simulink model "Wind_turbin."  (R2022b)
settings: Solver=ode45  StartTime=0.0  StopTime=Tsim  FixedStep=5e-5  RelTol=1e-6  EnableMultiTasking=on
values from neighbouring files (symbols this model uses):
  c1 = 0.44    [wind_code.m]
  c2 = 125    [wind_code.m]
  c3 = 0    [wind_code.m]
  c4 = 0    [wind_code.m]
  c5 = 0    [wind_code.m]
  c6 = 6.94    [wind_code.m]
  c7 = 16.5    [wind_code.m]
  c8 = 0    [wind_code.m]
  c9 = -0.002    [wind_code.m]
  N = 80    [wind_code.m]
  p = 2    [wind_code.m]
undefined symbols (not defined in the file or in its folder): A, Cdc, f_n1, fluxm, Jtot, Kcp, ki_dc, ki_m, ki_P_n1, ki_pll_n1, ki_s_n1, kp_dc, kp_md, kp_mq, kp_P_n1, kp_pll_n1, kp_s_n1, Lc_n1, Ld, Lg_n1, Lq, magnitud_delay, pitch, Q_set, Rc_n1, Rg_n1, rho, Rs, Rt, t_step_Q, Vdcref_n1, Vpeak_n1, w_n1
libraries: spsControlledVoltageSourceLib x9, slpidlib x8, spsSeriesRLCBranchLib x7, spsCurrentMeasurementLib x3, spsGroundLib x2, spsThreePhaseVIMeasurementLib x2, spsControlledCurrentSourceLib x2, spsPower3phInstantaneousLib x2, spsPermanentMagnetSynchronousMachineLib x1, spsVoltageMeasurementLib x1, sps_lib x1
(part 1 of 2)
settings Model: ExtModeTrigDuration=100  Creator=Enric  LastModifiedBy=Admin
settings SolverCC: SolverJacobianMethodControl=FullPerturbation  AlgebraicLoopSolver=TrustRegion
settings DataIOCC: LimitDataPoints=on  SaveOutput=off  ReturnWorkspaceOutputs=off  StateSaveName=tmp_raccel_xout  SignalLoggingName=tmp_raccel_logsout
settings OptimizationCC: ReuseModelBlockBuffer=on  EfficientMapNaN2IntZero=off  LifeSpan=inf
settings DebuggingCC: UnconnectedInputMsg=warning  UnconnectedOutputMsg=warning  UnconnectedLineMsg=warning  AllowSymbolicDim=off  SFUnexpectedBacktrackingDiag=warning  SFNoUnconditionalDefaultTransitionDiag=warning  SFExecutionAtInitializationDiag=none  ArithmeticOperatorsInVariantConditions=warning
settings HardwareCC: TargetBitPerPointer=64  TargetBitPerSizeT=64  TargetBitPerPtrDiffT=64  TargetLongLongMode=on  TargetIntDivRoundTo=Zero  TargetEndianess=LittleEndian  TargetWordSize=64  TargetHWDeviceType=MATLAB Host  ProdEqTarget=off
settings ModelReferenceCC: EnableRefExpFcnMdlSchedulingChecks=on  PropagateSignalLabelsOutOfModel=off
settings SFSimCC: SimUseLocalCustomCode=off  CustomCodeUndefinedFunction=UseInterfaceOnly
settings RTWCC: SystemTargetFile=raccel.tlc  TemplateMakefile=raccel_default_tmf  RTWVerbose=off  RTWUseLocalCustomCode=off  RTWUseSimCustomCode=on  DLArmComputeVersion=19.05
settings CodeAppCC: GenerateComments=off  MaxIdLength=128  MangleLength=10  SimulinkBlockComments=off
settings RaccelTargetCC: OptimizeReductions=off  ENABLE_SLEXEC_SSBRIDGE=0  RTWCAPISignals=off  RTWCAPIParams=on  RTWCAPIRootIO=off
settings ConfigComp: CovMetricSettings=dw  CovSaveCumulativeToWorkspaceVar=on  CovSaveSingleToWorkspaceVar=on  CovExternalEMLEnable=off
settings SimscapeCC: SimscapeNormalizeSystem=off

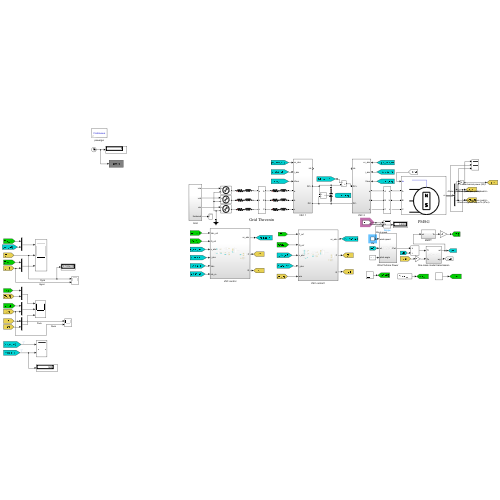
[thumbnail: Simulink's stored preview of the top-level diagram]
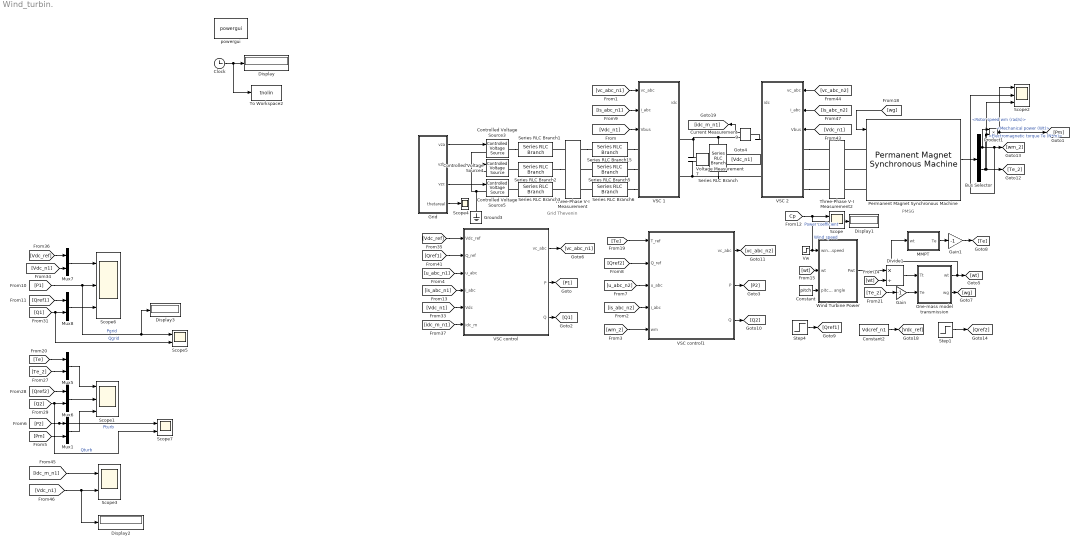
== system Wind_turbin. ==
  note: Grid Thevenin
  note: PMSG
  Bus Selector : BusSelector  OutputSignals=Rotor speed wm (rad/s),Electromagnetic torque Te (N*m)
  Clock : Clock
  Constant : Constant  Value=pitch
  Constant2 : Constant  Value=Vdcref_n1
  Controlled Voltage Source3 : spsControlledVoltageSourceLib/Controlled Voltage Source  Initialize=off  Source_Type=AC  Amplitude=0  Phase=0  Frequency=0  Measurements=None
  Controlled Voltage Source4 : spsControlledVoltageSourceLib/Controlled Voltage Source  Initialize=off  Source_Type=AC  Amplitude=0  Phase=0  Frequency=0  Measurements=None
  Controlled Voltage Source5 : spsControlledVoltageSourceLib/Controlled Voltage Source  Initialize=off  Source_Type=AC  Amplitude=0  Phase=0  Frequency=0  Measurements=None
  Current Measurement9 : spsCurrentMeasurementLib/Current Measurement  PhasorSimulation=off  OutputType=Complex  PSBequivalent=0
  Display{,1..3} (4 alike) : Display
  Divide1 : Product  Inputs=*/
  Gain : Gain  Gain=-1
  Gain1 : Gain  Gain=-1
  Grid : Subsystem
  Ground3 : spsGroundLib/Ground  LConnTagsString=a
  MMPT : Subsystem
  Mux{1,5..8} (5 alike) : Mux  Inputs=2
  One-mass model transmission : Subsystem
  Permanent Magnet Synchronous Machine : spsPermanentMagnetSynchronousMachineLib/Permanent Magnet Synchronous Machine  NbPhases=3  FluxDistribution=Sinusoidal  RotorType=Round  MechanicalLoad=Speed w  PresetModel=No  ShowDetailedParameters=on  MeasurementBus=off  Resistance=Rs  Inductance=8.5e-3  dqInductances=[Ld,Lq]  La=Lqd  MachineConstant=Flux linkage established by magnets (V.s)  Flux=fluxm  VoltageCst=906.8997  TorqueCst=7.5  Flat=120  Mechanical=[0.0027 0 1 0]  PolePairs=p  InitialConditions=[w_n1/p,0, 0,0]  InitialConditions5ph=[0 0 0 0 0 0]  RefAngle=90 degrees behind phase A axis (modified Park)  IterativeDiscreteModel=Trapezoidal non iterative  TsBlock=-1  TsPowergui=0
  Product1 : Product
  Scope{,3,5,7} (4 alike) : Scope  NumInputPorts=2
  Scope1 : Scope  NumInputPorts=3
  Scope2 : Scope  NumInputPorts=3
  Scope4 : Scope
  Scope6 : Scope  NumInputPorts=3
  Series RLC Branch : spsSeriesRLCBranchLib/Series RLC Branch  LConnTagsString=__new0  RConnTagsString=__new0  BranchType=C  Resistance=1  Inductance=1e-3  SetiL0=off  InitialCurrent=0  Capacitance=Cdc  Setx0=on  InitialVoltage=Vdcref_n1  Measurements=None
  Series RLC Branch1 : spsSeriesRLCBranchLib/Series RLC Branch  LConnTagsString=__new0  RConnTagsString=__new0  BranchType=RL  Resistance=Rg_n1  Inductance=Lg_n1  SetiL0=off  InitialCurrent=0  Capacitance=0  Setx0=off  InitialVoltage=0  Measurements=None
  Series RLC Branch15 : spsSeriesRLCBranchLib/Series RLC Branch  LConnTagsString=__new0  RConnTagsString=__new0  BranchType=RL  Resistance=Rc_n1  Inductance=Lc_n1  SetiL0=off  InitialCurrent=0  Capacitance=0  Setx0=off  InitialVoltage=0  Measurements=None
  Series RLC Branch2 : spsSeriesRLCBranchLib/Series RLC Branch  LConnTagsString=__new0  RConnTagsString=__new0  BranchType=RL  Resistance=Rg_n1  Inductance=Lg_n1  SetiL0=off  InitialCurrent=0  Capacitance=0  Setx0=off  InitialVoltage=0  Measurements=None
  Series RLC Branch3 : spsSeriesRLCBranchLib/Series RLC Branch  LConnTagsString=__new0  RConnTagsString=__new0  BranchType=RL  Resistance=Rg_n1  Inductance=Lg_n1  SetiL0=off  InitialCurrent=0  Capacitance=0  Setx0=off  InitialVoltage=0  Measurements=None
  Series RLC Branch5 : spsSeriesRLCBranchLib/Series RLC Branch  LConnTagsString=__new0  RConnTagsString=__new0  BranchType=RL  Resistance=Rc_n1  Inductance=Lc_n1  SetiL0=off  InitialCurrent=0  Capacitance=0  Setx0=off  InitialVoltage=0  Measurements=None
  Series RLC Branch6 : spsSeriesRLCBranchLib/Series RLC Branch  LConnTagsString=__new0  RConnTagsString=__new0  BranchType=RL  Resistance=Rc_n1  Inductance=Lc_n1  SetiL0=off  InitialCurrent=0  Capacitance=0  Setx0=off  InitialVoltage=0  Measurements=None
  Step1 : Step  Time=t_step_Q  After=0  SampleTime=0
  Step4 : Step  Time=t_step_Q  Before=Q_set  After=Q_set*1.2  SampleTime=0
  Three-Phase V-I Measurement : spsThreePhaseVIMeasurementLib/Three-Phase V-I Measurement  VoltageMeasurement=phase-to-ground  SetLabelV=on  LabelV=u_abc_n1  Vpu=off  VpuLL=off  CurrentMeasurement=yes  SetLabelI=on  LabelI=is_abc_n1  Ipu=off  Pbase=100e6  Vbase=500e3  OutputType=Complex  PhasorSimulation=off  PSBequivalent=0
  Three-Phase V-I Measurement2 : spsThreePhaseVIMeasurementLib/Three-Phase V-I Measurement  VoltageMeasurement=phase-to-ground  SetLabelV=on  LabelV=u_abc_n2  Vpu=off  VpuLL=off  CurrentMeasurement=yes  SetLabelI=on  LabelI=is_abc_n2  Ipu=off  Pbase=100e6  Vbase=500e3  OutputType=Complex  PhasorSimulation=off  PSBequivalent=0
  To Workspace2 : ToWorkspace  VariableName=tnolin  SampleTime=-1
  VSC 1 : Subsystem
  VSC 2 : Subsystem
  VSC control : Subsystem
  VSC control1 : Subsystem
  Voltage Measurement7 : spsVoltageMeasurementLib/Voltage Measurement  PhasorSimulation=off  OutputType=Complex  PSBequivalent=0
  Vw : Step  Time=0.5  Before=5  After=8  SampleTime=0
  Wind Turbine Power : Subsystem
  powergui : sps_lib/powergui  Priority=1  SimulationMode=Continuous  SampleTime=1e-5  frequency=60  Iterations=50  frequencyindice=0  Pbase=100e6  ErrMax=1e-4  UnitsV=kV  UnitsW=MW  buscounter=0  FunctionMessages=off  echomessages=off  EnableUseOfTLC=off  CurrentSourceSwitches=off  DisableSnubberDevices=off  DisableRonSwitches=off  DisableVfSwitches=off  DisplayEquations=off  AutomaticDiscreteSolvers=off  SolverType=Tustin  Interpol=off  ExternalGateDelay=off  methode=off  Ts=0  x0status=blocks  SPID=off  SwTol=0  HookPort=off  NonlinearTolerance=1e-4  nMaxIteration=100  ContinueOnMaxIteration=off  RestoreLinks=warning  ResistiveCurrentMeasurement=off  Frange=[0:2:500]  Ylog=off  Xlog=on  ShowGrid=off  save=off  variable=ZData  structure=Vk  ZoomFFT=off  StartTime=2.01  cycles=3  DisplayStyle=1  fundamental=50  FreqAxis=off  MaxFrequency=1000  frequencyindicesteady=1  RmsSteady=1  display=off
  wires:
  Clock/1 -> To Workspace2/1, Display/1
  [Vdc_n1] -> VSC 1/3(Vbus)
  [is_abc_n1] -> VSC 1/2(i_abc)
  [vc_abc_n1] -> VSC 1/1(vc_abc)
  Voltage Measurement7/1 -> [Vdc_n1]
  Grid/1(vza) -> Controlled Voltage Source3/1
  Grid/3(vzc) -> Controlled Voltage Source5/1
  Grid/4(thetareal) -> Scope4/1
  Grid/2(vzb) -> Controlled Voltage Source4/1
  Step4/1 -> [Qref1]
  Mux6/1 -> Scope1/2
  Mux5/1 -> Scope1/1
  [Qref2] -> Mux6/1
  [Te_2] -> Mux5/2
  [Q2] -> Scope7/2, Mux6/2  "Qturb"
  [Vdc_n1] -> Mux7/2
  [Vdc_ref] -> Mux7/1
  Mux7/1 -> Scope6/1
  [P1] -> Display3/1, Scope5/1, Scope6/2  "Pgrid"
  [Q1] -> Scope5/2, Mux8/2  "Qgrid"
  [Qref1] -> Mux8/1
  Mux8/1 -> Scope6/3
  Current Measurement9/1 -> [idc_m_n1]
  [idc_m_n1] -> Scope3/1
  [Vdc_n1] -> Display2/1, Scope3/2
  Constant2/1 -> [Vdc_ref]
  Permanent Magnet Synchronous Machine/1 -> Bus Selector/1
  Bus Selector/1 -> Scope2/2, [wm_2], Product1/1  "<Rotor speed wm (rad/s)>"
  Bus Selector/2 -> [Te_2], Scope2/3, Product1/2  "<Electromagnetic torque Te (N*m)>"
  [Vdc_n1] -> VSC 2/3(Vbus)
  [is_abc_n2] -> VSC 2/2(i_abc)
  [vc_abc_n2] -> VSC 2/1(vc_abc)
  [Vdc_ref] -> VSC control/1(Vdc_ref)
  [Qref1] -> VSC control/2(Q_ref)
  VSC control/1(vc_abc) -> [vc_abc_n1]
  [u_abc_n1] -> VSC control/3(u_abc)
  [is_abc_n1] -> VSC control/4(i_abc)
  [Vdc_n1] -> VSC control/5(Vdc)
  [idc_m_n1] -> VSC control/6(idc_m)
  VSC control/2(P) -> [P1]
  VSC control/3(Q) -> [Q1]
  [is_abc_n2] -> VSC control1/4(i_abc)
  [u_abc_n2] -> VSC control1/3(u_abc)
  [Qref2] -> VSC control1/2(Q_ref)
  VSC control1/3(Q) -> [Q2]
  VSC control1/1(vc_abc) -> [vc_abc_n2]
  VSC control1/2(P) -> [P2]
  [wm_2] -> VSC control1/5(wm)
  Product1/1 -> Scope2/1, [Pm]  "<Mechanical power (Wt)>"
  [Pm] -> Mux1/2
  Mux1/1 -> Scope1/3
  [P2] -> Scope7/1, Mux1/1  "Pturb"
  One-mass model transmission/2(wg) -> [wg]
  [wt] -> Wind Turbine Power/2(wt)
  Wind Turbine Power/1(Pwt) -> Divide1/1
  One-mass model transmission/1(wt) -> MMPT/1(wt), [wt]
  MMPT/1(Te) -> Gain1/1
  [wt] -> Divide1/2
  Constant/1 -> Wind Turbine Power/3(pitch angle)
  Divide1/1 -> One-mass model transmission/1(Tt)
  Gain/1 -> One-mass model transmission/2(Te)
  [Te_2] -> Gain/1
  [wg] -> Permanent Magnet Synchronous Machine/1
  Vw/1 -> Scope/2, Wind Turbine Power/1(wind speed)  "Wind speed"
  [Te] -> VSC control1/1(T_ref)
  Gain1/1 -> [Te]
  [Te] -> Mux5/1
  Step1/1 -> [Qref2]
  [Cp] -> Display1/1, Scope/1  "Power coefficient"
  connections:
  Series RLC Branch6/RConn1 -- VSC 1/LConn3
  Series RLC Branch15/RConn1 -- VSC 1/LConn1
  Series RLC Branch5/RConn1 -- VSC 1/LConn2
  Three-Phase V-I Measurement/LConn1 -- Series RLC Branch15/LConn1
  Series RLC Branch6/LConn1 -- Three-Phase V-I Measurement/LConn3
  Series RLC Branch5/LConn1 -- Three-Phase V-I Measurement/LConn2
  Controlled Voltage Source5/LConn1 -- Ground3/LConn1 -- Controlled Voltage Source3/LConn1 -- Controlled Voltage Source4/LConn1
  Controlled Voltage Source3/RConn1 -- Series RLC Branch1/LConn1
  Series RLC Branch2/LConn1 -- Controlled Voltage Source4/RConn1
  Series RLC Branch3/LConn1 -- Controlled Voltage Source5/RConn1
  Three-Phase V-I Measurement/RConn3 -- Series RLC Branch3/RConn1
  Voltage Measurement7/LConn1 -- Current Measurement9/RConn1 -- Series RLC Branch/LConn1 -- VSC 1/RConn1
  Voltage Measurement7/LConn2 -- VSC 2/RConn2 -- Series RLC Branch/RConn1 -- VSC 1/RConn2
  Series RLC Branch2/RConn1 -- Three-Phase V-I Measurement/RConn2
  Three-Phase V-I Measurement/RConn1 -- Series RLC Branch1/RConn1
  VSC 2/LConn1 -- Three-Phase V-I Measurement2/LConn1
  VSC 2/LConn2 -- Three-Phase V-I Measurement2/LConn2
  VSC 2/LConn3 -- Three-Phase V-I Measurement2/LConn3
  Permanent Magnet Synchronous Machine/LConn1 -- Three-Phase V-I Measurement2/RConn1
  Permanent Magnet Synchronous Machine/LConn2 -- Three-Phase V-I Measurement2/RConn2
  Permanent Magnet Synchronous Machine/LConn3 -- Three-Phase V-I Measurement2/RConn3
  VSC 2/RConn1 -- Current Measurement9/LConn1

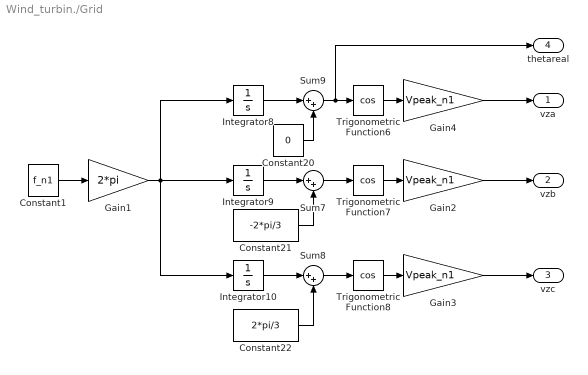
== system Wind_turbin./Grid ==
  Constant1 : Constant  Value=f_n1
  Constant20 : Constant  Value=0
  Constant21 : Constant  Value=-2*pi/3
  Constant22 : Constant  Value=2*pi/3
  Gain1 : Gain  Gain=2*pi
  Gain2 : Gain  Gain=Vpeak_n1
  Gain3 : Gain  Gain=Vpeak_n1
  Gain4 : Gain  Gain=Vpeak_n1
  Integrator10 : Integrator
  Integrator8 : Integrator
  Integrator9 : Integrator
  Sum7 : Sum  Inputs=|++
  Sum8 : Sum  Inputs=|++
  Sum9 : Sum  Inputs=|++
  Trigonometric Function6 : Trigonometry  Operator=cos
  Trigonometric Function7 : Trigonometry  Operator=cos
  Trigonometric Function8 : Trigonometry  Operator=cos
  vza : Outport
  vzb : Outport  Port=2
  vzc : Outport  Port=3
  thetareal : Outport  Port=4
  wires:
  Trigonometric Function7/1 -> Gain2/1
  Trigonometric Function8/1 -> Gain3/1
  Constant1/1 -> Gain1/1
  Sum9/1 -> thetareal/1, Trigonometric Function6/1
  Constant22/1 -> Sum8/2
  Integrator10/1 -> Sum8/1
  Constant21/1 -> Sum7/2
  Integrator8/1 -> Sum9/1
  Gain1/1 -> Integrator8/1, Integrator9/1, Integrator10/1
  Sum7/1 -> Trigonometric Function7/1
  Constant20/1 -> Sum9/2
  Trigonometric Function6/1 -> Gain4/1
  Integrator9/1 -> Sum7/1
  Sum8/1 -> Trigonometric Function8/1
  Gain4/1 -> vza/1
  Gain2/1 -> vzb/1
  Gain3/1 -> vzc/1

== system Wind_turbin./MMPT ==
  wt : Inport
  Gain6 : Gain  Gain=Kcp/N
  Product : Product
  Te : Outport
  wires:
  Product/1 -> Gain6/1
  wt/1 -> Product/1, Product/2
  Gain6/1 -> Te/1

== system Wind_turbin./One-mass model transmission ==
  Tt : Inport
  Te : Inport  Port=2
  Gain2 : Gain  Gain=N
  Gain3 : Gain  Gain=1/Jtot
  Gain4 : Gain  Gain=N
  Integrator : Integrator  InitialCondition=1
  Sum : Sum  Inputs=+-
  wt : Outport
  wg : Outport  Port=2
  wires:
  Gain4/1 -> wg/1
  Sum/1 -> Gain3/1
  Integrator/1 -> Gain4/1, wt/1
  Tt/1 -> Sum/1
  Gain3/1 -> Integrator/1
  Gain2/1 -> Sum/2
  Te/1 -> Gain2/1

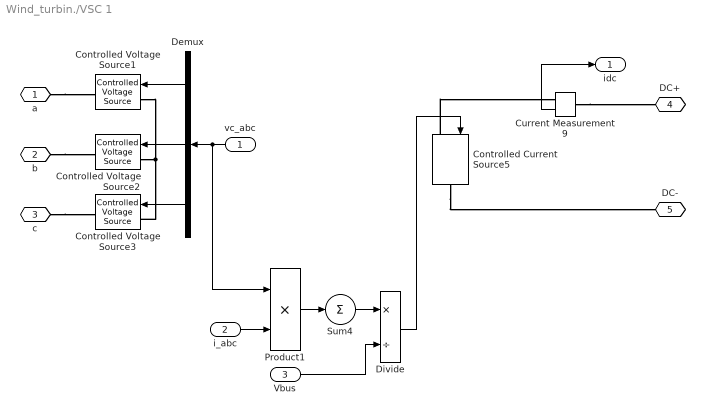
== system Wind_turbin./VSC 1 ==
  vc_abc : Inport
  i_abc : Inport  Port=2
  Vbus : Inport  Port=3
  Controlled Current Source5 : spsControlledCurrentSourceLib/Controlled Current Source  Initialize=on  Source_Type=DC  Amplitude=0  Phase=0  Frequency=0  Measurements=None
  Controlled Voltage Source1 : spsControlledVoltageSourceLib/Controlled Voltage Source  Initialize=off  Source_Type=AC  Amplitude=0  Phase=0  Frequency=0  Measurements=None
  Controlled Voltage Source2 : spsControlledVoltageSourceLib/Controlled Voltage Source  Initialize=off  Source_Type=AC  Amplitude=0  Phase=0  Frequency=0  Measurements=None
  Controlled Voltage Source3 : spsControlledVoltageSourceLib/Controlled Voltage Source  Initialize=off  Source_Type=AC  Amplitude=0  Phase=0  Frequency=0  Measurements=None
  Current Measurement9 : spsCurrentMeasurementLib/Current Measurement  PhasorSimulation=off  OutputType=Complex  PSBequivalent=0
  Demux : Demux  Outputs=3
  Divide : Product  Inputs=*/
  Product1 : Product  InputSameDT=on  SaturateOnIntegerOverflow=on  OutDataTypeStr=Inherit: Same as first input
  Sum4 : Sum  Inputs=1  InputSameDT=on  SaturateOnIntegerOverflow=on  OutDataTypeStr=Inherit: Same as first input
  a : PMIOPort  Side=Left
  b : PMIOPort  Port=2  Side=Left
  c : PMIOPort  Port=3  Side=Left
  DC+ : PMIOPort  Port=4  Side=Right
  DC- : PMIOPort  Port=5  Side=Right
  idc : Outport
  wires:
  Current Measurement9/1 -> idc/1
  Product1/1 -> Sum4/1
  Sum4/1 -> Divide/1
  Divide/1 -> Controlled Current Source5/1
  i_abc/1 -> Product1/2
  Demux/2 -> Controlled Voltage Source2/1
  Demux/1 -> Controlled Voltage Source1/1
  Demux/3 -> Controlled Voltage Source3/1
  vc_abc/1 -> Product1/1, Demux/1
  Vbus/1 -> Divide/2
  connections:
  Controlled Current Source5/RConn1 -- DC-/RConn1
  Controlled Current Source5/LConn1 -- Current Measurement9/RConn1
  Current Measurement9/LConn1 -- DC+/RConn1
  Controlled Voltage Source1/LConn1 -- Controlled Voltage Source2/LConn1 -- Controlled Voltage Source3/LConn1
  a/RConn1 -- Controlled Voltage Source1/RConn1
  b/RConn1 -- Controlled Voltage Source2/RConn1
  c/RConn1 -- Controlled Voltage Source3/RConn1

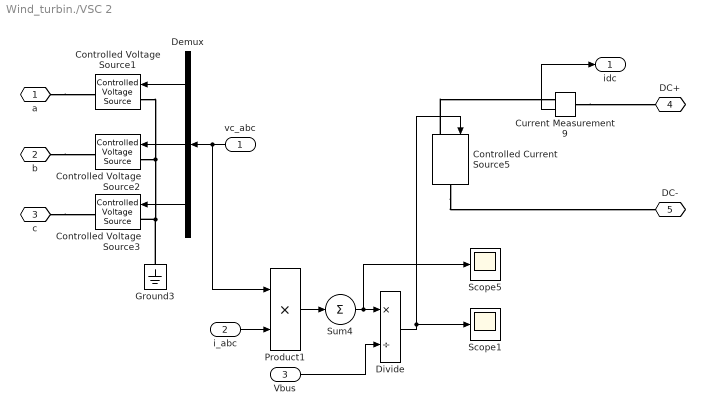
== system Wind_turbin./VSC 2 ==
  vc_abc : Inport
  i_abc : Inport  Port=2
  Vbus : Inport  Port=3
  Controlled Current Source5 : spsControlledCurrentSourceLib/Controlled Current Source  Initialize=on  Source_Type=DC  Amplitude=0  Phase=0  Frequency=0  Measurements=None
  Controlled Voltage Source1 : spsControlledVoltageSourceLib/Controlled Voltage Source  Initialize=off  Source_Type=AC  Amplitude=0  Phase=0  Frequency=0  Measurements=None
  Controlled Voltage Source2 : spsControlledVoltageSourceLib/Controlled Voltage Source  Initialize=off  Source_Type=AC  Amplitude=0  Phase=0  Frequency=0  Measurements=None
  Controlled Voltage Source3 : spsControlledVoltageSourceLib/Controlled Voltage Source  Initialize=off  Source_Type=AC  Amplitude=0  Phase=0  Frequency=0  Measurements=None
  Current Measurement9 : spsCurrentMeasurementLib/Current Measurement  PhasorSimulation=off  OutputType=Complex  PSBequivalent=0
  Demux : Demux  Outputs=3
  Divide : Product  Inputs=*/
  Ground3 : spsGroundLib/Ground  LConnTagsString=a
  Product1 : Product  InputSameDT=on  SaturateOnIntegerOverflow=on  OutDataTypeStr=Inherit: Same as first input
  Scope1 : Scope
  Scope5 : Scope
  Sum4 : Sum  Inputs=1  InputSameDT=on  SaturateOnIntegerOverflow=on  OutDataTypeStr=Inherit: Same as first input
  a : PMIOPort  Side=Left
  b : PMIOPort  Port=2  Side=Left
  c : PMIOPort  Port=3  Side=Left
  DC+ : PMIOPort  Port=4  Side=Right
  DC- : PMIOPort  Port=5  Side=Right
  idc : Outport
  wires:
  Current Measurement9/1 -> idc/1
  Product1/1 -> Sum4/1
  Sum4/1 -> Scope5/1, Divide/1
  Divide/1 -> Scope1/1, Controlled Current Source5/1
  i_abc/1 -> Product1/2
  Demux/2 -> Controlled Voltage Source2/1
  Demux/1 -> Controlled Voltage Source1/1
  Demux/3 -> Controlled Voltage Source3/1
  vc_abc/1 -> Product1/1, Demux/1
  Vbus/1 -> Divide/2
  connections:
  Controlled Current Source5/RConn1 -- DC-/RConn1
  Controlled Current Source5/LConn1 -- Current Measurement9/RConn1
  Current Measurement9/LConn1 -- DC+/RConn1
  Controlled Voltage Source1/LConn1 -- Controlled Voltage Source2/LConn1 -- Ground3/LConn1 -- Controlled Voltage Source3/LConn1
  a/RConn1 -- Controlled Voltage Source1/RConn1
  b/RConn1 -- Controlled Voltage Source2/RConn1
  c/RConn1 -- Controlled Voltage Source3/RConn1

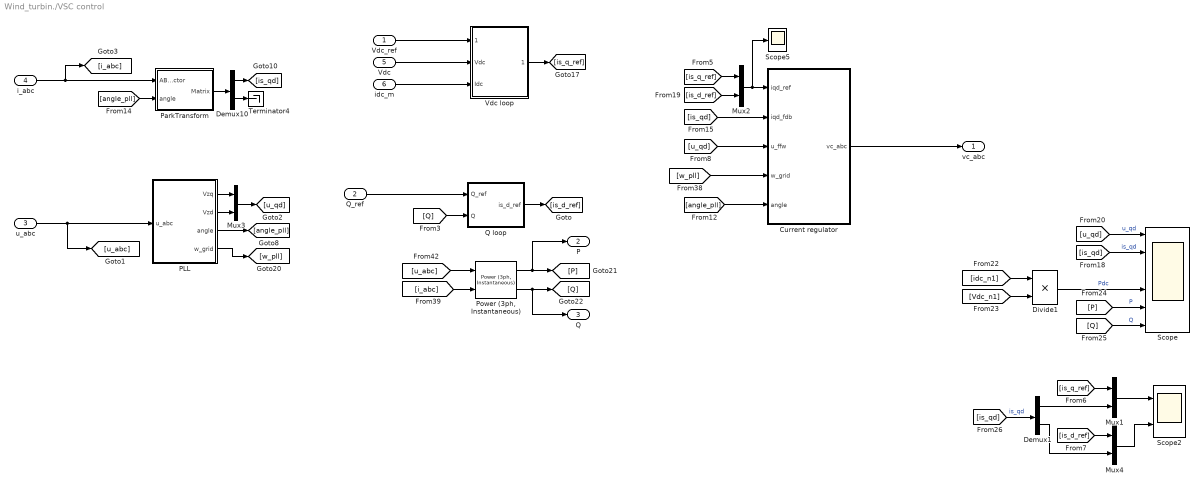
== system Wind_turbin./VSC control ==
  Vdc_ref : Inport
  Q_ref : Inport  Port=2
  u_abc : Inport  Port=3
  i_abc : Inport  Port=4
  Vdc : Inport  Port=5
  idc_m : Inport  Port=6
  Current regulator : Subsystem
  Demux1 : Demux  Outputs=2
  Demux10 : Demux  Outputs=2
  Divide1 : Product  Inputs=**
  Mux{1..4} (4 alike) : Mux  Inputs=2
  PLL : Subsystem
  ParkTransform : Subsystem  mask(Gerard){}
      mask help:
      | This block applies the park transfomation from a desired vector.
      | The input Xabc refers to the vector in the ABC frame, and the second input is the angle used in the transformation.
      | The output is the vector in the qd0 frame.
      mask Display:
      | port_label('output',1,'Xqd0')
      | port_label('input',1,'Xabc')
      | port_label('input',2,'angle')
  "Power (3ph, Instantaneous)" : spsPower3phInstantaneousLib/Power (3ph, Instantaneous)
  Q loop : Subsystem
  Scope : Scope  NumInputPorts=6
  Scope2 : Scope  NumInputPorts=2
  Scope5 : Scope
  Terminator4 : Terminator
  Vdc loop : Subsystem
  vc_abc : Outport
  P : Outport  Port=2
  Q : Outport  Port=3
  wires:
  Mux2/1 -> Scope5/1, Current regulator/1(iqd_ref)
  [is_d_ref] -> Mux2/2
  [w_pll] -> Current regulator/4(w_grid)
  PLL/4(w_grid) -> [w_pll]
  [is_qd] -> Current regulator/2(iqd_fdb)
  Q_ref/1 -> Q loop/1(Q_ref)
  PLL/3(angle) -> [angle_pll]
  PLL/2(Vzd) -> Mux3/2
  Demux10/1 -> [is_qd]
  Q loop/1(is_d_ref) -> [is_d_ref]
  PLL/1(Vzq) -> Mux3/1
  Current regulator/1(vc_abc) -> vc_abc/1
  ParkTransform/1(Matrix) -> Demux10/1
  i_abc/1 -> [i_abc], ParkTransform/1(ABC vector)
  Mux3/1 -> [u_qd]
  [u_qd] -> Current regulator/3(u_ffw)
  Demux10/2 -> Terminator4/1
  [is_q_ref] -> Mux2/1
  [angle_pll] -> Current regulator/5(angle)
  [u_abc] -> "Power (3ph, Instantaneous)"/1
  Vdc loop/1(is_q_ref) -> [is_q_ref]
  "Power (3ph, Instantaneous)"/1 -> P/1, [P]
  [Q] -> Q loop/2(Q)
  Vdc/1 -> Vdc loop/2(Vdc)
  [i_abc] -> "Power (3ph, Instantaneous)"/2
  idc_m/1 -> Vdc loop/3(Idc)
  [angle_pll] -> ParkTransform/2(angle)
  "Power (3ph, Instantaneous)"/2 -> Q/1, [Q]
  Vdc_ref/1 -> Vdc loop/1(Vdc_ref)
  [idc_n1] -> Divide1/1
  Divide1/1 -> Scope/4  "Pdc"
  [P] -> Scope/5  "P"
  [Vdc_n1] -> Divide1/2
  [u_qd] -> Scope/1  "u_qd"
  [is_qd] -> Scope/2  "is_qd"
  [Q] -> Scope/6  "Q"
  Demux1/1 -> Mux1/2
  [is_d_ref] -> Mux4/1
  Mux4/1 -> Scope2/2
  Mux1/1 -> Scope2/1
  Demux1/2 -> Mux4/2
  [is_qd] -> Demux1/1  "is_qd"
  [is_q_ref] -> Mux1/1
  u_abc/1 -> [u_abc], PLL/1(u_abc)

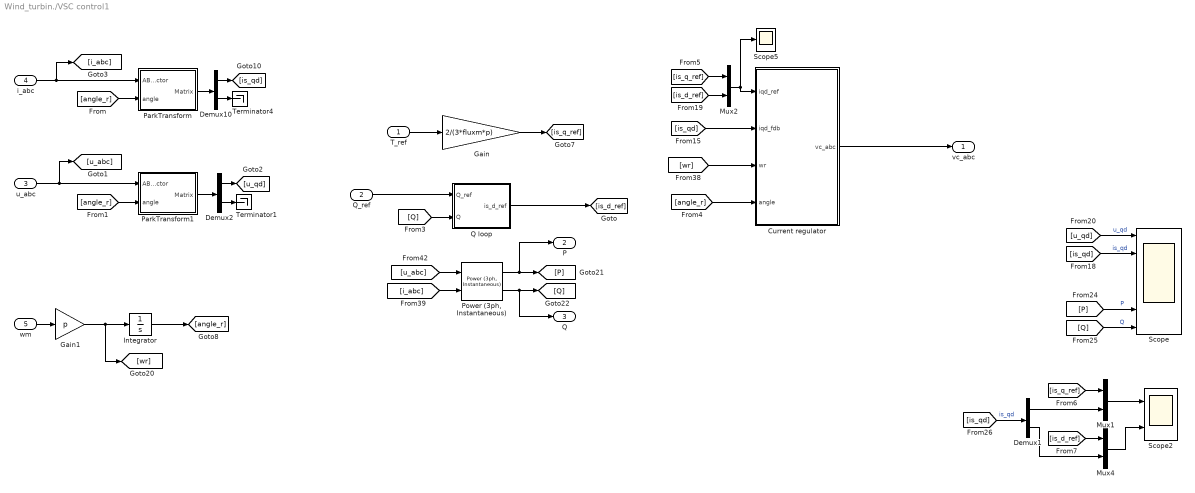
== system Wind_turbin./VSC control1 ==
  T_ref : Inport
  Q_ref : Inport  Port=2
  u_abc : Inport  Port=3
  i_abc : Inport  Port=4
  wm : Inport  Port=5
  Current regulator : Subsystem
  Demux1 : Demux  Outputs=2
  Demux10 : Demux  Outputs=2
  Demux2 : Demux  Outputs=2
  Gain : Gain  Gain=2/(3*fluxm*p)
  Gain1 : Gain  Gain=p
  Integrator : Integrator
  Mux1 : Mux  Inputs=2
  Mux2 : Mux  Inputs=2
  Mux4 : Mux  Inputs=2
  ParkTransform : Subsystem  mask(Gerard){}
      mask help:
      | This block applies the park transfomation from a desired vector.
      | The input Xabc refers to the vector in the ABC frame, and the second input is the angle used in the transformation.
      | The output is the vector in the qd0 frame.
      mask Display:
      | port_label('output',1,'Xqd0')
      | port_label('input',1,'Xabc')
      | port_label('input',2,'angle')
  ParkTransform1 : Subsystem  mask(Gerard){}
      mask help:
      | This block applies the park transfomation from a desired vector.
      | The input Xabc refers to the vector in the ABC frame, and the second input is the angle used in the transformation.
      | The output is the vector in the qd0 frame.
      mask Display:
      | port_label('output',1,'Xqd0')
      | port_label('input',1,'Xabc')
      | port_label('input',2,'angle')
  "Power (3ph, Instantaneous)" : spsPower3phInstantaneousLib/Power (3ph, Instantaneous)
  Q loop : Subsystem
  Scope : Scope  NumInputPorts=6
  Scope2 : Scope  NumInputPorts=2
  Scope5 : Scope
  Terminator1 : Terminator
  Terminator4 : Terminator
  vc_abc : Outport
  P : Outport  Port=2
  Q : Outport  Port=3
  wires:
  Mux2/1 -> Scope5/1, Current regulator/1(iqd_ref)
  [is_d_ref] -> Mux2/2
  [wr] -> Current regulator/3(wr)
  wm/1 -> Gain1/1
  [is_qd] -> Current regulator/2(iqd_fdb)
  Q_ref/1 -> Q loop/1(Q_ref)
  Integrator/1 -> [angle_r]
  Demux10/1 -> [is_qd]
  Current regulator/1(vc_abc) -> vc_abc/1
  ParkTransform/1(Matrix) -> Demux10/1
  i_abc/1 -> [i_abc], ParkTransform/1(ABC vector)
  Demux10/2 -> Terminator4/1
  [is_q_ref] -> Mux2/1
  [angle_r] -> Current regulator/4(angle)
  [u_abc] -> "Power (3ph, Instantaneous)"/1
  "Power (3ph, Instantaneous)"/1 -> P/1, [P]
  Gain/1 -> [is_q_ref]
  [Q] -> Q loop/2(Q)
  [i_abc] -> "Power (3ph, Instantaneous)"/2
  [angle_r] -> ParkTransform/2(angle)
  "Power (3ph, Instantaneous)"/2 -> Q/1, [Q]
  T_ref/1 -> Gain/1
  [P] -> Scope/5  "P"
  [u_qd] -> Scope/1  "u_qd"
  [is_qd] -> Scope/2  "is_qd"
  [Q] -> Scope/6  "Q"
  Demux1/1 -> Mux1/2
  [is_d_ref] -> Mux4/1
  Mux4/1 -> Scope2/2
  Mux1/1 -> Scope2/1
  Demux1/2 -> Mux4/2
  [is_qd] -> Demux1/1  "is_qd"
  [is_q_ref] -> Mux1/1
  u_abc/1 -> ParkTransform1/1(ABC vector), [u_abc]
  [angle_r] -> ParkTransform1/2(angle)
  Demux2/1 -> [u_qd]
  Demux2/2 -> Terminator1/1
  ParkTransform1/1(Matrix) -> Demux2/1
  Q loop/1(is_d_ref) -> [is_d_ref]
  Gain1/1 -> [wr], Integrator/1

== system Wind_turbin./Wind Turbine Power ==
  wind speed : Inport
  wt : Inport  Port=2
  pitch angle : Inport  Port=3
  Cp : Subsystem
  Divide : Product  Inputs=/*
  Gain : Gain  Gain=1/2*A*rho
  Gain1 : Gain  Gain=Rt
  Product : Product  Inputs=3
  Product1 : Product
  alfa : Subsystem
  Pwt : Outport
  tag scope: Cp=global
  wires:
  Gain/1 -> Product1/1
  wind speed/1 -> Divide/1, Product/1, Product/3, Product/2
  Divide/1 -> alfa/1(tip speed)
  Product/1 -> Gain/1
  Product1/1 -> Pwt/1
  wt/1 -> Gain1/1
  alfa/1(Out1) -> Cp/1(In1)
  Cp/1(Cp) -> [Cp], Product1/2
  pitch angle/1 -> Cp/2(pitch angle), alfa/2(pitch angle)
  Gain1/1 -> Divide/2

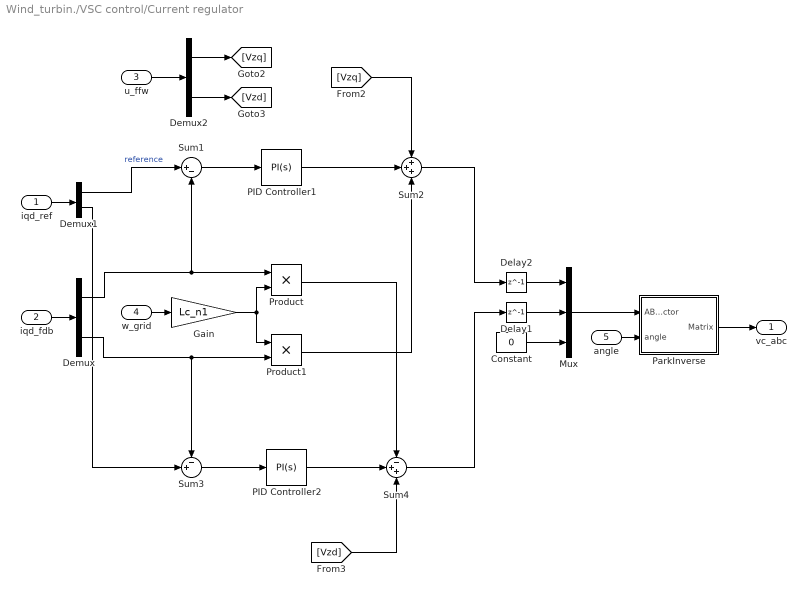
== system Wind_turbin./VSC control/Current regulator ==
  iqd_ref : Inport
  iqd_fdb : Inport  Port=2
  u_ffw : Inport  Port=3
  w_grid : Inport  Port=4
  angle : Inport  Port=5
  Constant : Constant  Value=0
  Delay1 : Delay  DelayLength=1  InitialCondition=0  SampleTime=magnitud_delay
  Delay2 : Delay  DelayLength=1  InitialCondition=Vpeak_n1  SampleTime=magnitud_delay
  Demux : Demux  Outputs=2
  Demux1 : Demux  Outputs=2
  Demux2 : Demux  Outputs=2
  Gain : Gain  Gain=Lc_n1
  Mux : Mux  Inputs=3
  PID Controller1 : slpidlib/PID Controller  Controller=PI  Form=Parallel  TimeDomain=Continuous-time  UseExternalTs=off  SampleTime=-1  IntegratorMethod=Forward Euler  FilterMethod=Forward Euler  ControllerParametersSource=internal  P=kp_s_n1  I=ki_s_n1  UseKiTs=off  D=0  N=100  UseFilter=on  TunerSelectOption=Transfer Function Based (PID Tuner App)  InitialConditionSource=internal  InitialConditionForIntegrator=0  InitialConditionForFilter=0  DifferentiatorICPrevScaledInput=0  ExternalReset=none  TrackingMode=off  Kt=1  LimitOutput=off  SatLimitsSource=internal  UpperSaturationLimit=inf  LowerSaturationLimit=-inf  LinearizeAsGain=on  AntiWindupMode=none  Kb=1  LimitIntegrator=off  UpperIntegratorSaturationLimit=inf  LowerIntegratorSaturationLimit=-inf  POutMin=[]  POutMax=[]  IOutMin=[]  IOutMax=[]  DOutMin=[]  DOutMax=[]  NOutMin=[]  NOutMax=[]  SumOutMin=[]  SumOutMax=[]  SaturationOutMin=[]  SaturationOutMax=[]  PParamMin=[]  PParamMax=[]  IParamMin=[]  IParamMax=[]  DParamMin=[]  DParamMax=[]  NParamMin=[]  NParamMax=[]  KbParamMin=[]  KbParamMax=[]  KtParamMin=[]  KtParamMax=[]  KbOutMin=[]  KbOutMax=[]  KtOutMin=[]  KtOutMax=[]  IntegratorOutMin=[]  IntegratorOutMax=[]  FilterOutMin=[]  FilterOutMax=[]  SumI1OutMin=[]  SumI1OutMax=[]  SumI2OutMin=[]  SumI2OutMax=[]  SumI3OutMin=[]  SumI3OutMax=[]  SumI4OutMin=[]  SumI4OutMax=[]  SumDOutMin=[]  SumDOutMax=[]  DifferentiatorOutMin=[]  DifferentiatorOutMax=[]  FilterDiffOutCoefMin=[]  FilterDiffOutCoefMax=[]  ReciprocalOutMin=[]  ReciprocalOutMax=[]  SumDenOutMin=[]  SumDenOutMax=[]  SumNumOutMin=[]  SumNumOutMax=[]  DivideOutMin=[]  DivideOutMax=[]  UdiffTsProdOutMin=[]  UdiffTsProdOutMax=[]  NTsProdOutMin=[]  NTsProdOutMax=[]  UintegralTsProdOutMin=[]  UintegralTsProdOutMax=[]  UngainTsProdOutMin=[]  UngainTsProdOutMax=[]  ClampingZeroOutDataTypeStr=Inherit: Inherit via back propagation  ClampingZeroOutMin=[]  ClampingZeroOutMax=[]  FilterDenConstantOutDataTypeStr=Inherit: Inherit via back propagation  FilterDenConstantOutMin=[]  FilterDenConstantOutMax=[]  PCopyOutDataTypeStr=Inherit: Inherit via back propagation  PCopyOutMin=[]  PCopyOutMax=[]  NCopyOutDataTypeStr=Inherit: Inherit via back propagation  NCopyOutMin=[]  NCopyOutMax=[]  IntegratorContinuousStateAttributes=''  IntegratorStateMustResolveToSignalObject=off  IntegratorRTWStateStorageClass=Auto  FilterContinuousStateAttributes=''  FilterStateMustResolveToSignalObject=off  FilterRTWStateStorageClass=Auto  ParallelPVariant=InternalParameters  IdealPVariant=Disabled  IVariant=InternalParameters  DVariant=Disabled  IntegratorVariant=Continuous  SatVariant=Disabled  AWVariant=Passthrough  PCopyVariant=Disabled  TRVariant=Disabled  FdbkBlocksVariant=Forward  IdealPFdbkVariant=Disabled  SatFdbkVariant=Disabled  DerivativeFilterVariant=Disabled  NVariant=Disabled  NCopyVariant=Disabled_SignalSpec  FilterICVariant=Disabled  IntegratorICVariant=InternalICs  ExternalResetVariant=Disabled  TRSumVariant=Passthrough  SumFdbkVariant=Disabled  SumVariant=Sum_PI  TsampFilterVariant=InternalTs  TsampNgainVariant=Passthrough  TsampIntegralVariant=Passthrough  ExternalSaturationOutDataTypeStr=Inherit: Same as second input
  PID Controller2 : slpidlib/PID Controller  Controller=PI  Form=Parallel  TimeDomain=Continuous-time  UseExternalTs=off  SampleTime=-1  IntegratorMethod=Forward Euler  FilterMethod=Forward Euler  ControllerParametersSource=internal  P=kp_s_n1  I=ki_s_n1  UseKiTs=off  D=0  N=100  UseFilter=on  TunerSelectOption=Transfer Function Based (PID Tuner App)  InitialConditionSource=internal  InitialConditionForIntegrator=0  InitialConditionForFilter=0  DifferentiatorICPrevScaledInput=0  ExternalReset=none  TrackingMode=off  Kt=1  LimitOutput=off  SatLimitsSource=internal  UpperSaturationLimit=inf  LowerSaturationLimit=-inf  LinearizeAsGain=on  AntiWindupMode=none  Kb=1  LimitIntegrator=off  UpperIntegratorSaturationLimit=inf  LowerIntegratorSaturationLimit=-inf  POutMin=[]  POutMax=[]  IOutMin=[]  IOutMax=[]  DOutMin=[]  DOutMax=[]  NOutMin=[]  NOutMax=[]  SumOutMin=[]  SumOutMax=[]  SaturationOutMin=[]  SaturationOutMax=[]  PParamMin=[]  PParamMax=[]  IParamMin=[]  IParamMax=[]  DParamMin=[]  DParamMax=[]  NParamMin=[]  NParamMax=[]  KbParamMin=[]  KbParamMax=[]  KtParamMin=[]  KtParamMax=[]  KbOutMin=[]  KbOutMax=[]  KtOutMin=[]  KtOutMax=[]  IntegratorOutMin=[]  IntegratorOutMax=[]  FilterOutMin=[]  FilterOutMax=[]  SumI1OutMin=[]  SumI1OutMax=[]  SumI2OutMin=[]  SumI2OutMax=[]  SumI3OutMin=[]  SumI3OutMax=[]  SumI4OutMin=[]  SumI4OutMax=[]  SumDOutMin=[]  SumDOutMax=[]  DifferentiatorOutMin=[]  DifferentiatorOutMax=[]  FilterDiffOutCoefMin=[]  FilterDiffOutCoefMax=[]  ReciprocalOutMin=[]  ReciprocalOutMax=[]  SumDenOutMin=[]  SumDenOutMax=[]  SumNumOutMin=[]  SumNumOutMax=[]  DivideOutMin=[]  DivideOutMax=[]  UdiffTsProdOutMin=[]  UdiffTsProdOutMax=[]  NTsProdOutMin=[]  NTsProdOutMax=[]  UintegralTsProdOutMin=[]  UintegralTsProdOutMax=[]  UngainTsProdOutMin=[]  UngainTsProdOutMax=[]  ClampingZeroOutDataTypeStr=Inherit: Inherit via back propagation  ClampingZeroOutMin=[]  ClampingZeroOutMax=[]  FilterDenConstantOutDataTypeStr=Inherit: Inherit via back propagation  FilterDenConstantOutMin=[]  FilterDenConstantOutMax=[]  PCopyOutDataTypeStr=Inherit: Inherit via back propagation  PCopyOutMin=[]  PCopyOutMax=[]  NCopyOutDataTypeStr=Inherit: Inherit via back propagation  NCopyOutMin=[]  NCopyOutMax=[]  IntegratorContinuousStateAttributes=''  IntegratorStateMustResolveToSignalObject=off  IntegratorRTWStateStorageClass=Auto  FilterContinuousStateAttributes=''  FilterStateMustResolveToSignalObject=off  FilterRTWStateStorageClass=Auto  ParallelPVariant=InternalParameters  IdealPVariant=Disabled  IVariant=InternalParameters  DVariant=Disabled  IntegratorVariant=Continuous  SatVariant=Disabled  AWVariant=Passthrough  PCopyVariant=Disabled  TRVariant=Disabled  FdbkBlocksVariant=Forward  IdealPFdbkVariant=Disabled  SatFdbkVariant=Disabled  DerivativeFilterVariant=Disabled  NVariant=Disabled  NCopyVariant=Disabled_SignalSpec  FilterICVariant=Disabled  IntegratorICVariant=InternalICs  ExternalResetVariant=Disabled  TRSumVariant=Passthrough  SumFdbkVariant=Disabled  SumVariant=Sum_PI  TsampFilterVariant=InternalTs  TsampNgainVariant=Passthrough  TsampIntegralVariant=Passthrough  ExternalSaturationOutDataTypeStr=Inherit: Same as second input
  ParkInverse : Subsystem  mask(Gerard){}
      mask help:
      | This block applies the park inverse transfomation from a desired vector.
      | The input Xqd0 refers to the vector in the qd0 frame, and the second input is the angle used in the inverse transformation.
      | The output is the vector in the ABC frame.
      mask Display:
      | port_label('output',1,'Xabc')
      | port_label('input',1,'Xqd0')
      | port_label('input',2,'angle')
  Product : Product  RndMeth=Zero
  Product1 : Product  RndMeth=Zero
  Sum1 : Sum  Inputs=|+-
  Sum2 : Sum  Inputs=+++
  Sum3 : Sum  Inputs=-+|
  Sum4 : Sum  Inputs=-++
  vc_abc : Outport
  wires:
  iqd_fdb/1 -> Demux/1
  w_grid/1 -> Gain/1
  PID Controller1/1 -> Sum2/2
  Demux/1 -> Sum1/2, Product/1
  Gain/1 -> Product1/1, Product/2
  Demux/2 -> Product1/2, Sum3/1
  Product1/1 -> Sum2/3
  Product/1 -> Sum4/1
  Constant/1 -> Mux/3
  ParkInverse/1(Matrix) -> vc_abc/1
  iqd_ref/1 -> Demux1/1
  [Vzq] -> Sum2/1
  Mux/1 -> ParkInverse/1(ABC vector)
  Demux2/1 -> [Vzq]
  Demux2/2 -> [Vzd]
  u_ffw/1 -> Demux2/1
  [Vzd] -> Sum4/3
  angle/1 -> ParkInverse/2(angle)
  Sum1/1 -> PID Controller1/1
  Sum3/1 -> PID Controller2/1
  PID Controller2/1 -> Sum4/2
  Demux1/2 -> Sum3/2
  Demux1/1 -> Sum1/1  "reference"
  Sum4/1 -> Delay1/1
  Sum2/1 -> Delay2/1
  Delay1/1 -> Mux/2
  Delay2/1 -> Mux/1

== system Wind_turbin./VSC control/PLL ==
  u_abc : Inport
  Constant : Constant  Value=0
  Constant3 : Constant  Value=2*pi*f_n1
  Demux : Demux  Outputs=3
  Integrator : Integrator
  PID Controller : slpidlib/PID Controller  Controller=PI  Form=Parallel  TimeDomain=Continuous-time  UseExternalTs=off  SampleTime=-1  IntegratorMethod=Forward Euler  FilterMethod=Forward Euler  ControllerParametersSource=internal  P=kp_pll_n1  I=ki_pll_n1  UseKiTs=off  D=0  N=100  UseFilter=on  TunerSelectOption=Transfer Function Based (PID Tuner App)  InitialConditionSource=internal  InitialConditionForIntegrator=0  InitialConditionForFilter=0  DifferentiatorICPrevScaledInput=0  ExternalReset=none  TrackingMode=off  Kt=1  LimitOutput=off  SatLimitsSource=internal  UpperSaturationLimit=inf  LowerSaturationLimit=-inf  LinearizeAsGain=on  AntiWindupMode=none  Kb=1  LimitIntegrator=off  UpperIntegratorSaturationLimit=inf  LowerIntegratorSaturationLimit=-inf  POutMin=[]  POutMax=[]  IOutMin=[]  IOutMax=[]  DOutMin=[]  DOutMax=[]  NOutMin=[]  NOutMax=[]  SumOutMin=[]  SumOutMax=[]  SaturationOutMin=[]  SaturationOutMax=[]  PParamMin=[]  PParamMax=[]  IParamMin=[]  IParamMax=[]  DParamMin=[]  DParamMax=[]  NParamMin=[]  NParamMax=[]  KbParamMin=[]  KbParamMax=[]  KtParamMin=[]  KtParamMax=[]  KbOutMin=[]  KbOutMax=[]  KtOutMin=[]  KtOutMax=[]  IntegratorOutMin=[]  IntegratorOutMax=[]  FilterOutMin=[]  FilterOutMax=[]  SumI1OutMin=[]  SumI1OutMax=[]  SumI2OutMin=[]  SumI2OutMax=[]  SumI3OutMin=[]  SumI3OutMax=[]  SumI4OutMin=[]  SumI4OutMax=[]  SumDOutMin=[]  SumDOutMax=[]  DifferentiatorOutMin=[]  DifferentiatorOutMax=[]  FilterDiffOutCoefMin=[]  FilterDiffOutCoefMax=[]  ReciprocalOutMin=[]  ReciprocalOutMax=[]  SumDenOutMin=[]  SumDenOutMax=[]  SumNumOutMin=[]  SumNumOutMax=[]  DivideOutMin=[]  DivideOutMax=[]  UdiffTsProdOutMin=[]  UdiffTsProdOutMax=[]  NTsProdOutMin=[]  NTsProdOutMax=[]  UintegralTsProdOutMin=[]  UintegralTsProdOutMax=[]  UngainTsProdOutMin=[]  UngainTsProdOutMax=[]  ClampingZeroOutDataTypeStr=Inherit: Inherit via back propagation  ClampingZeroOutMin=[]  ClampingZeroOutMax=[]  FilterDenConstantOutDataTypeStr=Inherit: Inherit via back propagation  FilterDenConstantOutMin=[]  FilterDenConstantOutMax=[]  PCopyOutDataTypeStr=Inherit: Inherit via back propagation  PCopyOutMin=[]  PCopyOutMax=[]  NCopyOutDataTypeStr=Inherit: Inherit via back propagation  NCopyOutMin=[]  NCopyOutMax=[]  IntegratorContinuousStateAttributes=''  IntegratorStateMustResolveToSignalObject=off  IntegratorRTWStateStorageClass=Auto  FilterContinuousStateAttributes=''  FilterStateMustResolveToSignalObject=off  FilterRTWStateStorageClass=Auto  ParallelPVariant=InternalParameters  IdealPVariant=Disabled  IVariant=InternalParameters  DVariant=Disabled  IntegratorVariant=Continuous  SatVariant=Disabled  AWVariant=Passthrough  PCopyVariant=Disabled  TRVariant=Disabled  FdbkBlocksVariant=Forward  IdealPFdbkVariant=Disabled  SatFdbkVariant=Disabled  DerivativeFilterVariant=Disabled  NVariant=Disabled  NCopyVariant=Disabled_SignalSpec  FilterICVariant=Disabled  IntegratorICVariant=InternalICs  ExternalResetVariant=Disabled  TRSumVariant=Passthrough  SumFdbkVariant=Disabled  SumVariant=Sum_PI  TsampFilterVariant=InternalTs  TsampNgainVariant=Passthrough  TsampIntegralVariant=Passthrough  ExternalSaturationOutDataTypeStr=Inherit: Same as second input
  ParkTransform : Subsystem  mask(Gerard){}
      mask help:
      | This block applies the park transfomation from a desired vector.
      | The input Xabc refers to the vector in the ABC frame, and the second input is the angle used in the transformation.
      | The output is the vector in the qd0 frame.
      mask Display:
      | port_label('output',1,'Xqd0')
      | port_label('input',1,'Xabc')
      | port_label('input',2,'angle')
  Scope1 : Scope
  Scope2 : Scope
  Scope20 : Scope
  Sum : Sum  Inputs=|+-
  Sum1 : Sum  Inputs=|++
  Terminator8 : Terminator
  Vzq : Outport
  Vzd : Outport  Port=2
  angle : Outport  Port=3
  w_grid : Outport  Port=4
  wires:
  Constant3/1 -> Sum1/2
  Demux/2 -> Vzd/1, Sum/2
  Sum1/1 -> Scope1/1, w_grid/1, Integrator/1
  Constant/1 -> Sum/1
  Integrator/1 -> Scope2/1, ParkTransform/2(angle), angle/1
  Demux/3 -> Terminator8/1
  PID Controller/1 -> Sum1/1
  u_abc/1 -> ParkTransform/1(ABC vector)
  ParkTransform/1(Matrix) -> Demux/1
  Demux/1 -> Vzq/1
  Sum/1 -> PID Controller/1, Scope20/1

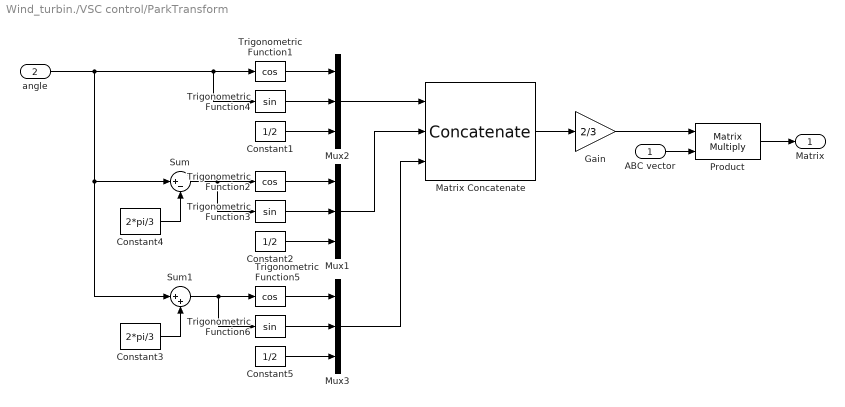
== system Wind_turbin./VSC control/ParkTransform ==
  ABC vector : Inport
  angle : Inport  Port=2
  Constant1 : Constant  Value=1/2
  Constant2 : Constant  Value=1/2
  Constant3 : Constant  Value=2*pi/3
  Constant4 : Constant  Value=2*pi/3
  Constant5 : Constant  Value=1/2
  Gain : Gain  Gain=2/3
  Matrix Concatenate : Concatenate  NumInputs=3  Mode=Multidimensional array  ConcatenateDimension=2
  Mux1 : Mux  Inputs=3
  Mux2 : Mux  Inputs=3
  Mux3 : Mux  Inputs=3
  Product : Product  Multiplication=Matrix(*)  RndMeth=Zero
  Sum : Sum  Inputs=|+-
  Sum1 : Sum  Inputs=|++
  Trigonometric Function1 : Trigonometry  Operator=cos
  Trigonometric Function2 : Trigonometry  Operator=cos
  Trigonometric Function3 : Trigonometry
  Trigonometric Function4 : Trigonometry
  Trigonometric Function5 : Trigonometry  Operator=cos
  Trigonometric Function6 : Trigonometry
  Matrix : Outport
  wires:
  Matrix Concatenate/1 -> Gain/1
  ABC vector/1 -> Product/2
  Product/1 -> Matrix/1
  Gain/1 -> Product/1
  Constant4/1 -> Sum/2
  Constant3/1 -> Sum1/2
  angle/1 -> Trigonometric Function4/1, Trigonometric Function1/1, Sum1/1, Sum/1
  Trigonometric Function3/1 -> Mux1/2
  Trigonometric Function2/1 -> Mux1/1
  Constant2/1 -> Mux1/3
  Sum/1 -> Trigonometric Function3/1, Trigonometric Function2/1
  Trigonometric Function4/1 -> Mux2/2
  Trigonometric Function1/1 -> Mux2/1
  Constant1/1 -> Mux2/3
  Trigonometric Function6/1 -> Mux3/2
  Trigonometric Function5/1 -> Mux3/1
  Constant5/1 -> Mux3/3
  Sum1/1 -> Trigonometric Function6/1, Trigonometric Function5/1
  Mux1/1 -> Matrix Concatenate/2
  Mux2/1 -> Matrix Concatenate/1
  Mux3/1 -> Matrix Concatenate/3

== system Wind_turbin./VSC control/Q loop ==
  Q_ref : Inport
  Q : Inport  Port=2
  Gain2 : Gain  Gain=2/(3*Vpeak_n1)
  PID Controller : slpidlib/PID Controller  Controller=PI  Form=Parallel  TimeDomain=Continuous-time  UseExternalTs=off  SampleTime=-1  IntegratorMethod=Forward Euler  FilterMethod=Forward Euler  ControllerParametersSource=internal  P=kp_P_n1  I=ki_P_n1  UseKiTs=off  D=0  N=100  UseFilter=on  TunerSelectOption=Transfer Function Based (PID Tuner App)  InitialConditionSource=internal  InitialConditionForIntegrator=0  InitialConditionForFilter=0  DifferentiatorICPrevScaledInput=0  ExternalReset=none  TrackingMode=off  Kt=1  LimitOutput=off  SatLimitsSource=internal  UpperSaturationLimit=inf  LowerSaturationLimit=-inf  LinearizeAsGain=on  AntiWindupMode=none  Kb=1  LimitIntegrator=off  UpperIntegratorSaturationLimit=inf  LowerIntegratorSaturationLimit=-inf  POutMin=[]  POutMax=[]  IOutMin=[]  IOutMax=[]  DOutMin=[]  DOutMax=[]  NOutMin=[]  NOutMax=[]  SumOutMin=[]  SumOutMax=[]  SaturationOutMin=[]  SaturationOutMax=[]  PParamMin=[]  PParamMax=[]  IParamMin=[]  IParamMax=[]  DParamMin=[]  DParamMax=[]  NParamMin=[]  NParamMax=[]  KbParamMin=[]  KbParamMax=[]  KtParamMin=[]  KtParamMax=[]  KbOutMin=[]  KbOutMax=[]  KtOutMin=[]  KtOutMax=[]  IntegratorOutMin=[]  IntegratorOutMax=[]  FilterOutMin=[]  FilterOutMax=[]  SumI1OutMin=[]  SumI1OutMax=[]  SumI2OutMin=[]  SumI2OutMax=[]  SumI3OutMin=[]  SumI3OutMax=[]  SumI4OutMin=[]  SumI4OutMax=[]  SumDOutMin=[]  SumDOutMax=[]  DifferentiatorOutMin=[]  DifferentiatorOutMax=[]  FilterDiffOutCoefMin=[]  FilterDiffOutCoefMax=[]  ReciprocalOutMin=[]  ReciprocalOutMax=[]  SumDenOutMin=[]  SumDenOutMax=[]  SumNumOutMin=[]  SumNumOutMax=[]  DivideOutMin=[]  DivideOutMax=[]  UdiffTsProdOutMin=[]  UdiffTsProdOutMax=[]  NTsProdOutMin=[]  NTsProdOutMax=[]  UintegralTsProdOutMin=[]  UintegralTsProdOutMax=[]  UngainTsProdOutMin=[]  UngainTsProdOutMax=[]  ClampingZeroOutDataTypeStr=Inherit: Inherit via back propagation  ClampingZeroOutMin=[]  ClampingZeroOutMax=[]  FilterDenConstantOutDataTypeStr=Inherit: Inherit via back propagation  FilterDenConstantOutMin=[]  FilterDenConstantOutMax=[]  PCopyOutDataTypeStr=Inherit: Inherit via back propagation  PCopyOutMin=[]  PCopyOutMax=[]  NCopyOutDataTypeStr=Inherit: Inherit via back propagation  NCopyOutMin=[]  NCopyOutMax=[]  IntegratorContinuousStateAttributes=''  IntegratorStateMustResolveToSignalObject=off  IntegratorRTWStateStorageClass=Auto  FilterContinuousStateAttributes=''  FilterStateMustResolveToSignalObject=off  FilterRTWStateStorageClass=Auto  ParallelPVariant=InternalParameters  IdealPVariant=Disabled  IVariant=InternalParameters  DVariant=Disabled  IntegratorVariant=Continuous  SatVariant=Disabled  AWVariant=Passthrough  PCopyVariant=Disabled  TRVariant=Disabled  FdbkBlocksVariant=Forward  IdealPFdbkVariant=Disabled  SatFdbkVariant=Disabled  DerivativeFilterVariant=Disabled  NVariant=Disabled  NCopyVariant=Disabled_SignalSpec  FilterICVariant=Disabled  IntegratorICVariant=InternalICs  ExternalResetVariant=Disabled  TRSumVariant=Passthrough  SumFdbkVariant=Disabled  SumVariant=Sum_PI  TsampFilterVariant=InternalTs  TsampNgainVariant=Passthrough  TsampIntegralVariant=Passthrough  ExternalSaturationOutDataTypeStr=Inherit: Same as second input
  Scope3 : Scope
  Sum1 : Sum  Inputs=|+-
  is_d_ref : Outport
  wires:
  Q_ref/1 -> Sum1/1
  Sum1/1 -> Scope3/1, PID Controller/1
  Q/1 -> Sum1/2
  PID Controller/1 -> Gain2/1
  Gain2/1 -> is_d_ref/1

== system Wind_turbin./VSC control/Vdc loop ==
  Vdc_ref : Inport
  Vdc : Inport  Port=2
  Idc : Inport  Port=3
  Gain1 : Gain  Gain=-1
  Gain2 : Gain  Gain=2/3*Vdcref_n1/Vpeak_n1
  Gain3 : Gain  Gain=0
  PID Controller : slpidlib/PID Controller  Controller=PI  Form=Parallel  TimeDomain=Continuous-time  UseExternalTs=off  SampleTime=-1  IntegratorMethod=Forward Euler  FilterMethod=Forward Euler  ControllerParametersSource=internal  P=kp_dc  I=ki_dc  UseKiTs=off  D=0  N=100  UseFilter=on  TunerSelectOption=Transfer Function Based (PID Tuner App)  InitialConditionSource=internal  InitialConditionForIntegrator=0  InitialConditionForFilter=0  DifferentiatorICPrevScaledInput=0  ExternalReset=none  TrackingMode=off  Kt=1  LimitOutput=off  SatLimitsSource=internal  UpperSaturationLimit=inf  LowerSaturationLimit=-inf  LinearizeAsGain=on  AntiWindupMode=none  Kb=1  LimitIntegrator=off  UpperIntegratorSaturationLimit=inf  LowerIntegratorSaturationLimit=-inf  POutMin=[]  POutMax=[]  IOutMin=[]  IOutMax=[]  DOutMin=[]  DOutMax=[]  NOutMin=[]  NOutMax=[]  SumOutMin=[]  SumOutMax=[]  SaturationOutMin=[]  SaturationOutMax=[]  PParamMin=[]  PParamMax=[]  IParamMin=[]  IParamMax=[]  DParamMin=[]  DParamMax=[]  NParamMin=[]  NParamMax=[]  KbParamMin=[]  KbParamMax=[]  KtParamMin=[]  KtParamMax=[]  KbOutMin=[]  KbOutMax=[]  KtOutMin=[]  KtOutMax=[]  IntegratorOutMin=[]  IntegratorOutMax=[]  FilterOutMin=[]  FilterOutMax=[]  SumI1OutMin=[]  SumI1OutMax=[]  SumI2OutMin=[]  SumI2OutMax=[]  SumI3OutMin=[]  SumI3OutMax=[]  SumI4OutMin=[]  SumI4OutMax=[]  SumDOutMin=[]  SumDOutMax=[]  DifferentiatorOutMin=[]  DifferentiatorOutMax=[]  FilterDiffOutCoefMin=[]  FilterDiffOutCoefMax=[]  ReciprocalOutMin=[]  ReciprocalOutMax=[]  SumDenOutMin=[]  SumDenOutMax=[]  SumNumOutMin=[]  SumNumOutMax=[]  DivideOutMin=[]  DivideOutMax=[]  UdiffTsProdOutMin=[]  UdiffTsProdOutMax=[]  NTsProdOutMin=[]  NTsProdOutMax=[]  UintegralTsProdOutMin=[]  UintegralTsProdOutMax=[]  UngainTsProdOutMin=[]  UngainTsProdOutMax=[]  ClampingZeroOutDataTypeStr=Inherit: Inherit via back propagation  ClampingZeroOutMin=[]  ClampingZeroOutMax=[]  FilterDenConstantOutDataTypeStr=Inherit: Inherit via back propagation  FilterDenConstantOutMin=[]  FilterDenConstantOutMax=[]  PCopyOutDataTypeStr=Inherit: Inherit via back propagation  PCopyOutMin=[]  PCopyOutMax=[]  NCopyOutDataTypeStr=Inherit: Inherit via back propagation  NCopyOutMin=[]  NCopyOutMax=[]  IntegratorContinuousStateAttributes=''  IntegratorStateMustResolveToSignalObject=off  IntegratorRTWStateStorageClass=Auto  FilterContinuousStateAttributes=''  FilterStateMustResolveToSignalObject=off  FilterRTWStateStorageClass=Auto  ParallelPVariant=InternalParameters  IdealPVariant=Disabled  IVariant=InternalParameters  DVariant=Disabled  IntegratorVariant=Continuous  SatVariant=Disabled  AWVariant=Passthrough  PCopyVariant=Disabled  TRVariant=Disabled  FdbkBlocksVariant=Forward  IdealPFdbkVariant=Disabled  SatFdbkVariant=Disabled  DerivativeFilterVariant=Disabled  NVariant=Disabled  NCopyVariant=Disabled_SignalSpec  FilterICVariant=Disabled  IntegratorICVariant=InternalICs  ExternalResetVariant=Disabled  TRSumVariant=Passthrough  SumFdbkVariant=Disabled  SumVariant=Sum_PI  TsampFilterVariant=InternalTs  TsampNgainVariant=Passthrough  TsampIntegralVariant=Passthrough  ExternalSaturationOutDataTypeStr=Inherit: Same as second input
  Scope3 : Scope
  Sum1 : Sum  Inputs=|+-
  Sum2 : Sum  Inputs=|+-
  is_q_ref : Outport
  wires:
  Sum1/1 -> Scope3/1, PID Controller/1
  Vdc_ref/1 -> Sum1/1
  Vdc/1 -> Sum1/2
  Gain1/1 -> Gain2/1
  Gain2/1 -> is_q_ref/1
  PID Controller/1 -> Sum2/1
  Sum2/1 -> Gain1/1
  Idc/1 -> Gain3/1
  Gain3/1 -> Sum2/2
